simulink model "Sums"  (R2023a)
settings: Solver=VariableStepAuto  StartTime=0.0  StopTime=10.0  RelTol=1e-3
settings Model: Creator=Ilya_Andriyanov  LastModifiedBy=Ilya_Andriyanov

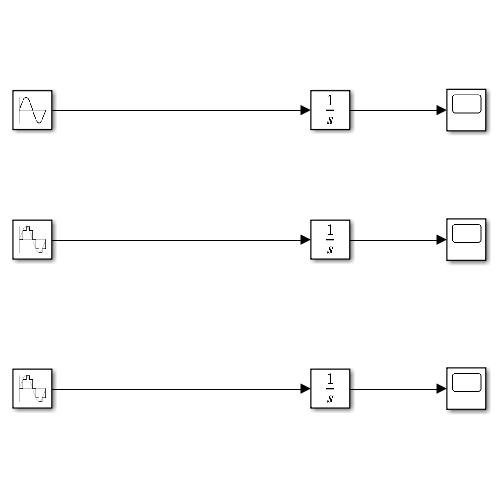
[thumbnail: Simulink's stored preview of the top-level diagram]
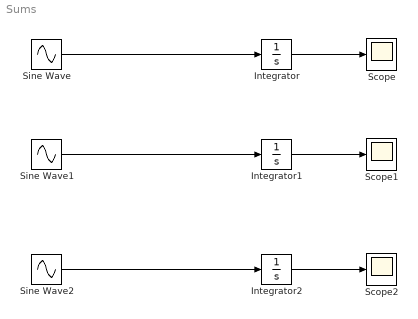
== system Sums ==
  Integrator : Integrator
  Integrator1 : Integrator
  Integrator2 : Integrator
  Scope : Scope
  Scope1 : Scope
  Scope2 : Scope
  Sine Wave : Sin  SampleTime=0
  Sine Wave1 : Sin  SampleTime=1
  Sine Wave2 : Sin  SampleTime=2
  wires:
  Sine Wave/1 -> Integrator/1
  Integrator/1 -> Scope/1
  Integrator1/1 -> Scope1/1
  Integrator2/1 -> Scope2/1
  Sine Wave1/1 -> Integrator1/1
  Sine Wave2/1 -> Integrator2/1
